simulink model "CAVE_MachE_dSPACE_250912"  (R2024a)
settings: configuration reference "ConfigSetDesktopFixedStep" (kept outside this file)
PreLoadFcn:
  | VSS_BICYCLE=Simulink.Variant('Dual=0');
  | VSS_DUAL=Simulink.Variant('Dual=1');
  | Dual=1;
  | load('DriveCycle2.mat')
PostLoadFcn:
  | if any(exist('dsrtsu_mdlpostloadfcn', 'file') ~= 0), dsrtsu_mdlpostloadfcn('Execute', bdroot); end
InitFcn:
  | , if any(exist('rtifpga_mdlclblib', 'file') ~= 0), rtifpga_mdlclblib('Init', bdroot); end,
  | , if any(exist('dsmpb_private', 'file') ~= 0), dsmpb_private('dsmpb_mdlclblib', 'Init', bdroot); end,
  | load('DriveCycle2.mat')
model workspace (MAT data in the model file):
  Gas = 0.383333333333
values from neighbouring files (symbols this model uses):
  CoastDown =     [Run_Simulink.mat]
  limitedMCT =     [Run_Simulink.mat]
  MCT =     [Run_Simulink.mat]
  pMCT =     [Run_Simulink.mat]
  RealSimPara =     [Run_Simulink.mat]
  Ref_speed = [13 13.007895099 13.015778396 13.023649891 13.031509584 13.039357475 13.047193564 13.055017851 13.062830336 13.070631019 13.0784199 13.086196979 ... (2669 elements, 2669x1)]    [Ref_speed_and_time.mat]
  Ref_time = [0 0.01 0.02 0.03 0.04 0.05 0.06 0.07 0.08 0.09 0.1 0.11 ... (2669 elements, 2669x1)]    [Ref_speed_and_time.mat]
  US06 =     [Run_Simulink.mat]
undefined symbols (not defined in the file or in its folder): AccelCmd, ActTqLF_Nm_, ActTqLR_Nm_, ActTqRF_Nm_, ActTqRR_Nm_, BattChargeLimitMaxPwr, BattChargeLimitSocBpts, BattChargeLimitTbl, BattChrgCapcty, BattDischargeLimitSocBpts, BattDischargeLimitTbl, BattDischargeMaxPwr, BattNumCellsParallel, BattNumCellsSeries, BattOpenVoltCapBpts, BattOpenVoltTbl, BattResistSocBpts, BattResistTbl, BattResistTempBpts, BrakeMaxPrs, BrakeMaxTrq, ChassisDistCg2FrontAxle, ChassisDistCg2RearAxle, ChassisVehMass, CltchCmd, DecelCmd, DiffRatio, DiscIntNeverNeededParam, EnvGravCnst, EnvPrs, EnvTemp, FuelSpecificGrav, GearCmd, h, InitStates, lgSw, MtrEffSpdBpts, MtrEffTbl, MtrEffTrqBpts, MtrPwrMax, MtrTrqMax, SteeringCmd, SupvsryCtrlRegenBrkCutOffTbl, SupvsryCtrlRegenSpdBpts, TestScnrioCycleNum, VEH
libraries: VSIGenLib x122, simulink x112, etargetslib x75, dsmpblib x55, vehdynlibtire x24, CarMaker4SL x20, autolibshared x19, vehdynlibsuspension x14, vehdynlibtirecommon x14, autolibutils x10, VsrLibWheel x8, autolibpowerinfoutils x6
(part 11 of 31)

== system CAVE_MachE_dSPACE_250912/Vehicle Under Test2/Vehicle/Vehicle Dynamics/Vehicle 14DOF/Wheel Routing1 ==
  Info : Inport
  Wheel : Inport  Port=2
  Bus Selector : BusSelector  OutputSignals=InertFrm.FrntAxl.Lft.Disp.Y,InertFrm.FrntAxl.Rght.Disp.Y,InertFrm.RearAxl.Lft.Disp.Y,InertFrm.RearAxl.Rght.Disp.Y
  Bus Selector1 : BusSelector  OutputSignals=InertFrm.FrntAxl.Lft.Disp.X,InertFrm.FrntAxl.Rght.Disp.X,InertFrm.RearAxl.Lft.Disp.X,InertFrm.RearAxl.Rght.Disp.X
  Bus Selector2 : BusSelector  OutputSignals=TireFrame.z,TireFrame.Omega,TireFrame.Kappa,TireFrame.Alpha
  Bus Selector3 : BusSelector  OutputSignals=InertFrm.FrntAxl.Lft.Disp.Z,InertFrm.FrntAxl.Rght.Disp.Z,InertFrm.RearAxl.Lft.Disp.Z,InertFrm.RearAxl.Rght.Disp.Z
  Bus Selector4 : BusSelector  OutputSignals=BdyFrm.FrntAxl.Lft.Disp.z,BdyFrm.FrntAxl.Rght.Disp.z,BdyFrm.RearAxl.Lft.Disp.z,BdyFrm.RearAxl.Rght.Disp.z
  Scope : Scope
  Scope1 : Scope
  Subtract : Sum  Inputs=-+-
  Vector Concatenate{1..4} (4 alike) : Concatenate  NumInputs=4
  Omega : Outport  PortDimensions=4  VectorParamsAs1DForOutWhenUnconnected=off
  Kappa : Outport  Port=2  PortDimensions=4  VectorParamsAs1DForOutWhenUnconnected=off
  Alpha : Outport  Port=3  PortDimensions=4  VectorParamsAs1DForOutWhenUnconnected=off
  XWheel : Outport  Port=4  Unit=m  VectorParamsAs1DForOutWhenUnconnected=off
  YWheel : Outport  Port=5  Unit=m  VectorParamsAs1DForOutWhenUnconnected=off
  ZWheel : Outport  Port=6  PortDimensions=4  VectorParamsAs1DForOutWhenUnconnected=off
  wires:
  Bus Selector4/2 -> Vector Concatenate4/2  "<z>"
  Bus Selector4/3 -> Vector Concatenate4/3  "<z>"
  Bus Selector4/4 -> Vector Concatenate4/4  "<z>"
  Bus Selector4/1 -> Vector Concatenate4/1  "<z>"
  Vector Concatenate4/1 -> Subtract/1
  Vector Concatenate3/1 -> Subtract/2
  Bus Selector3/1 -> Vector Concatenate3/1  "<Z>"
  Bus Selector3/4 -> Vector Concatenate3/4  "<Z>"
  Bus Selector3/3 -> Vector Concatenate3/3  "<Z>"
  Bus Selector3/2 -> Vector Concatenate3/2  "<Z>"
  Info/1 -> Bus Selector/1, Bus Selector3/1, Bus Selector4/1, Bus Selector1/1
  Subtract/1 -> ZWheel/1
  Wheel/1 -> Bus Selector2/1
  Bus Selector2/4 -> Alpha/1  "<Alpha>"
  Bus Selector2/3 -> Kappa/1  "<Kappa>"
  Bus Selector2/2 -> Scope/1, Omega/1  "<Omega>"
  Bus Selector2/1 -> Scope1/1, Subtract/3  "<z>"
  Vector Concatenate2/1 -> XWheel/1
  Bus Selector1/1 -> Vector Concatenate2/1  "<X>"
  Vector Concatenate1/1 -> YWheel/1
  Bus Selector/2 -> Vector Concatenate1/2  "<Y>"
  Bus Selector/3 -> Vector Concatenate1/3  "<Y>"
  Bus Selector1/2 -> Vector Concatenate2/2  "<X>"
  Bus Selector/4 -> Vector Concatenate1/4  "<Y>"
  Bus Selector1/3 -> Vector Concatenate2/3  "<X>"
  Bus Selector/1 -> Vector Concatenate1/1  "<Y>"
  Bus Selector1/4 -> Vector Concatenate2/4  "<X>"

== system CAVE_MachE_dSPACE_250912/Vehicle Under Test2/Vehicle/Vehicle Dynamics/Vehicle 14DOF/Wheels and Tires ==
  Suspension : Inport
  Axle Torque : Inport  Port=2
  Brake Press : Inport  Port=3  Unit=Pa
  Ground Input : Inport  Port=4
  Friction : Inport  Port=5  PortDimensions=4
  Bus Selector1 : BusSelector  OutputSignals=Whl.Ang,Whl.F,Whl.AngVel,Whl.xdot,Whl.ydot
  Constant3 : Constant  Value=zeros(4,1)
  Cont LPF : autolibutils/Cont LPF  wc=100*2*pi  AbsoluteTolerance=auto  aMode=2
  Cont LPF1 : autolibutils/Cont LPF  wc=100*2*pi  AbsoluteTolerance=auto  aMode=2
  Manual Switch6 : ManualSwitch
  Matrix Concatenate : Concatenate  NumInputs=3  Mode=Multidimensional array
  Reshape1 : Reshape
  Reshape2 : Reshape
  Saturation : Saturate  UpperLimit=10*9.81*2040  LowerLimit=-10*9.81*2040  ZeroCross=off
  Selector : Selector  NumberOfDimensions=2  InputPortWidth=3  IndexOptions=Index vector (dialog),Select all  Indices=[3],1  OutputSizes=1,1
  Selector1 : Selector  NumberOfDimensions=2  InputPortWidth=1  IndexOptions=Index vector (dialog),Select all  Indices=[3],1  OutputSizes=1,1
  Selector2 : Selector  NumberOfDimensions=2  InputPortWidth=3  IndexOptions=Index vector (dialog),Select all  Indices=3,1  OutputSizes=1,1
  Selector3 : Selector  NumberOfDimensions=2  InputPortWidth=3  IndexOptions=Index vector (dialog),Select all  Indices=1,1  OutputSizes=1,1
  Terminator{,1,3..5} (5 alike) : Terminator
  VDBS : Subsystem  VariantControl=0
  Wheels : Outport  VectorParamsAs1DForOutWhenUnconnected=off
  wires:
  VDBS/1(Wheels) -> Wheels/1  "Wheels"
  Bus Selector1/2 -> Selector/1  "<F>"
  VDBS/2(FrntAxlF) -> Terminator/1
  VDBS/3(RearAxlF) -> Terminator1/1
  VDBS/4(Omega) -> Terminator3/1
  VDBS/5(Mz) -> Terminator4/1
  Selector1/1 -> Reshape1/1
  Matrix Concatenate/1 -> VDBS/7(VehVel)
  Axle Torque/1 -> VDBS/3(AxleTrq)
  Selector2/1 -> VDBS/1(WheelAng)  "Wheel Angles"
  Constant3/1 -> Manual Switch6/1
  Manual Switch6/1 -> VDBS/2(CamberAng)  "Camber Angles"
  Selector/1 -> Reshape2/1
  Saturation/1 -> VDBS/5(Fz)
  Ground Input/1 -> VDBS/8(Ground Level)
  VDBS/7(SuspWhlVz) -> Matrix Concatenate/3  "zdot"
  Bus Selector1/1 -> Cont LPF1/1  "<Ang>"
  Selector3/1 -> Manual Switch6/2  "Camber Angles"
  Suspension/1 -> Bus Selector1/1
  Bus Selector1/4 -> Matrix Concatenate/1  "<xdot>"
  Bus Selector1/5 -> Matrix Concatenate/2  "<ydot>"
  VDBS/6(SuspWhlPz) -> Terminator5/1  "z"
  Reshape2/1 -> Cont LPF/1
  Bus Selector1/3 -> Selector1/1  "<AngVel>"
  Reshape1/1 -> VDBS/6(r)
  Brake Press/1 -> VDBS/4(BrkPrs)
  Friction/1 -> VDBS/9(Friction)
  Cont LPF/1 -> Saturation/1
  Cont LPF1/1 -> Selector3/1, Selector2/1

== system CAVE_MachE_dSPACE_250912/Vehicle Under Test2/Vehicle/Vehicle Dynamics/Vehicle 7DOF/Brake Pressure ==
  BrkReq : Inport
  Bus Creator1 : BusCreator  Inputs=2
  Gain : Gain  Gain=BrakeMaxPrs
  Gain{1..4} (4 alike) : Gain  Gain=0.5
  Saturation{,1..3} (4 alike) : Saturate  UpperLimit=BrakeMaxPrs  LowerLimit=0  ZeroCross=off
  Signal Specification : SignalSpecification  Unit=Pa
  Terminator : Terminator
  Vector Concatenate2 : Concatenate  NumInputs=4
  BrakePrs : Outport  Unit=Pa
  wires:
  BrkReq/1 -> Gain/1, Bus Creator1/1  "BrkReq"
  Gain/1 -> Signal Specification/1
  Signal Specification/1 -> Gain2/1, Gain1/1, Bus Creator1/2  "BrkPrs"
  Bus Creator1/1 -> Terminator/1  "WhlBrk"
  Gain1/1 -> Gain4/1
  Gain2/1 -> Gain3/1
  Gain3/1 -> Saturation/1, Saturation1/1
  Gain4/1 -> Saturation2/1, Saturation3/1
  Vector Concatenate2/1 -> BrakePrs/1
  Saturation/1 -> Vector Concatenate2/1
  Saturation1/1 -> Vector Concatenate2/2
  Saturation2/1 -> Vector Concatenate2/3
  Saturation3/1 -> Vector Concatenate2/4

== system CAVE_MachE_dSPACE_250912/Vehicle Under Test2/Vehicle/Vehicle Dynamics/Vehicle 7DOF/Longitudinal Wheels 4DOF ==
  WhlAng : Inport
  AxlTrq : Inport  Port=2
  BrkPrs : Inport  Port=3
  Gnd : Inport  Port=4  PortDimensions=4
  lam_mu : Inport  Port=5  PortDimensions=4
  VehFdbk : Inport  Port=6
  Axle Forces : Subsystem  Variant=on  VariantControlMode=label  LabelModeActiveChoice=1
  Bus Selector5 : BusSelector  OutputSignals=BdyFrm.Cg.AngVel.r
  Constant : vehdynlibtirecommon/Constant  const=220000  numWheels=4
  Constant3 : vehdynlibtirecommon/Constant  const=0  numWheels=4
  Terminator2 : Terminator
  Tire2Veh : Subsystem
  Tires : Subsystem
  Veh2Tire : Subsystem
  Velocity and Vertical Load : Subsystem  Variant=on  VariantControlMode=label  LabelModeActiveChoice=1
  Wheel Angles : Subsystem
  FrntAxlF : Outport  Unit=N  VectorParamsAs1DForOutWhenUnconnected=off
  RearAxlF : Outport  Port=2  Unit=N  VectorParamsAs1DForOutWhenUnconnected=off
  Omega : Outport  Port=3  VectorParamsAs1DForOutWhenUnconnected=off
  Kappa : Outport  Port=4  VectorParamsAs1DForOutWhenUnconnected=off
  Alpha : Outport  Port=5  VectorParamsAs1DForOutWhenUnconnected=off
  zAxle : Outport  Port=6  VectorParamsAs1DForOutWhenUnconnected=off
  wires:
  Wheel Angles/1(WhlAngB) -> Veh2Tire/5(WhlAng)
  Tires/1(Wheel) -> Tire2Veh/1(Wheel)
  lam_mu/1 -> Tires/9(lam_mu)
  Constant/1 -> Tires/7(TirePrs)
  Constant3/1 -> Wheel Angles/2(Camber), Tires/6(Camber)
  Veh2Tire/3(xdotAxle) -> Tires/3(Vx)  "Vx"
  Gnd/1 -> Tires/10(Gnd)
  VehFdbk/1 -> Bus Selector5/1, Velocity and Vertical Load/1(VehFdbk)
  AxlTrq/1 -> Veh2Tire/1(AxlTrq)
  Veh2Tire/1(T) -> Tires/1(AxlTrq)
  Veh2Tire/2(P) -> Tires/2(BrkPrs)
  BrkPrs/1 -> Veh2Tire/2(BrkPrs)
  Bus Selector5/1 -> Veh2Tire/3(r)  "<r>"
  Veh2Tire/6(zdotAxle) -> Terminator2/1
  WhlAng/1 -> Wheel Angles/1(WheelAng)  "FrontWheelAngles"
  Veh2Tire/4(ydotAxle) -> Tires/4(Vy)  "Vy"
  Veh2Tire/5(psidot) -> Tires/5(r)
  Velocity and Vertical Load/2(Fz) -> Tires/8(Fz)
  Velocity and Vertical Load/1(VehVel) -> Veh2Tire/4(VehVel)
  Axle Forces/1(FrntAxlF) -> FrntAxlF/1
  Axle Forces/2(RearAxlF) -> RearAxlF/1
  Tire2Veh/1(FwF) -> Axle Forces/1(F)
  Tire2Veh/2(FwR) -> Axle Forces/2(R)
  Tire2Veh/3(z) -> zAxle/1
  Tire2Veh/4(Omega) -> Omega/1
  Tire2Veh/5(Kappa) -> Kappa/1
  Tire2Veh/6(Alpha) -> Alpha/1

== system CAVE_MachE_dSPACE_250912/Vehicle Under Test2/Vehicle/Vehicle Dynamics/Vehicle 7DOF/RototestDummy ==
  Bus Creator1 : BusCreator  Inputs=ActTqLF_Nm_,ActTqRF_Nm_,ActTqLR_Nm_,ActTqRR_Nm_
  Bus Creator2 : BusCreator  Inputs=Car Trq_T2WFL,Car Trq_T2WFR,Car Trq_T2WRL,Car Trq_T2WRR
  Bus Creator3 : BusCreator  Inputs=1
  Bus Creator4 : BusCreator  Inputs=1
  Bus Selector14 : BusSelector  OutputSignals=VehSpd
  Bus Selector15 : BusSelector  OutputSignals=TireFrame.Fx
  Constant{1..14} (14 alike) : Constant  Value=0
  Vector Concatenate3 : Concatenate  NumInputs=4
  CarTrqT2W : Outport
  AxleTrq : Outport  Port=2
  BrakePressed_flag : Outport  Port=3
  <VehSpd> : Outport  Port=4
  <Fx> : Outport  Port=5
  wires:
  Constant10/1 -> Bus Selector14/1  "VehSpd"
  Bus Creator4/1 -> Bus Creator3/1  "TireFrame"
  Bus Creator1/1 -> AxleTrq/1  "AxleTrq"
  Constant9/1 -> Bus Creator1/4  "ActTqRR_Nm_"
  Constant13/1 -> Bus Creator2/3  "CarTrq_T2WRL"
  Constant4/1 -> Vector Concatenate3/4
  Bus Creator3/1 -> Bus Selector15/1
  Vector Concatenate3/1 -> Bus Creator4/1  "Fx"
  Constant3/1 -> Vector Concatenate3/3
  Constant2/1 -> Vector Concatenate3/2
  Constant14/1 -> Bus Creator2/4  "CarTrq_T2WRR"
  Constant6/1 -> Bus Creator1/1  "ActTqLF_Nm_"
  Constant1/1 -> Vector Concatenate3/1
  Constant8/1 -> Bus Creator1/3  "ActTqLR_Nm_"
  Constant11/1 -> Bus Creator2/1  "CarTrq_T2WFL"
  Constant7/1 -> Bus Creator1/2  "ActTqRF_Nm_"
  Constant12/1 -> Bus Creator2/2  "CarTrq_T2WFR"
  Bus Creator2/1 -> CarTrqT2W/1  "CarTrqT2W"
  Bus Selector14/1 -> <VehSpd>/1  "<VehSpd>"
  Constant5/1 -> BrakePressed_flag/1  "BrakePressed_flag"
  Bus Selector15/1 -> <Fx>/1  "<Fx>"

== system CAVE_MachE_dSPACE_250912/Vehicle Under Test2/Vehicle/Vehicle Dynamics/Vehicle 7DOF/Steering ==
  SteeringCmd : Inport
  Ground : Ground
  Kinematic Steering : vehdynlibsteering/Kinematic Steering  StrgType=Ackerman  StrgRatioType=Constant  Loc=Front  NrmlFctr=1  TrckWdth=1.9  WhlBase=ChassisDistCg2FrontAxle+ChassisDistCg2RearAxle  Db=0  StrgRng=3*pi  StrgAngBpts="[-6.2832   -5.0265   -3.7699   -2.5133   -1.2566         0    1.2566    2.5133    3.7699    5.0265    6.2832]"  StrgRatioTbl=|  StrgRatio=18  PctAckIn=off  PctAck=100  PctAckTbl=ones(1,11)*100  StrgArmLngth=0.1  RckCsLngth=0.5  TieRodLngth=0.248  D=0.2  PnnRadius=0.0057  PnnRadiusTbl="[0.0055    0.0055    0.0056    0.0057    0.0058    0.0057    0.0057    0.0057    0.0056    0.0055    0.0055]"  RodLngth=0.1  ParaArmLngth=0.9  aMode=2
      | [13.5000   13.3750   13.2500   13.1250   13.0000   13.0000   13.0000   13.1250   13.2500   13.3750   13.5000
      | ]
  Terminator1 : Terminator
  Vector Concatenate : Concatenate
  Vector Concatenate1 : Concatenate
  Vector Concatenate2 : Concatenate
  WhlAng : Outport  Unit=rad
  wires:
  Kinematic Steering/1 -> Terminator1/1
  Vector Concatenate2/1 -> WhlAng/1
  Kinematic Steering/2 -> Vector Concatenate/1
  Vector Concatenate1/1 -> Vector Concatenate2/2  "RearWheelAngles"
  Vector Concatenate/1 -> Vector Concatenate2/1  "FrontWheelAngles"
  Ground/1 -> Vector Concatenate1/2, Vector Concatenate1/1
  Kinematic Steering/3 -> Vector Concatenate/2
  SteeringCmd/1 -> Kinematic Steering/1

== system CAVE_MachE_dSPACE_250912/Vehicle Under Test2/Vehicle/Vehicle Dynamics/Vehicle 7DOF/Subsystem4 ==
  Cgxyzdot : Inport
  CgXYZ : Inport  Port=2
  CgXYZdot : Inport  Port=3
  angles : Inport  Port=4
  pqr : Inport  Port=5
  Cgaxyz : Inport  Port=6
  Beta : Inport  Port=7
  GeomXYZ : Inport  Port=8
  GeomXYZdot : Inport  Port=9
  Omega : Inport  Port=10
  Kappa : Inport  Port=11
  Alpha : Inport  Port=12
  XWheel : Inport  Port=13
  YWheel : Inport  Port=14
  dzWheel : Inport  Port=15
  Bus Creator : BusCreator  Inputs=26
  Bus Creator3 : BusCreator  Inputs=6
  Demux{,1..7} (8 alike) : Demux  Outputs=3
  Subsystem : Subsystem
  Chassis : Outport  VectorParamsAs1DForOutWhenUnconnected=off
  Wheels : Outport  Port=2  VectorParamsAs1DForOutWhenUnconnected=off
  wires:
  Bus Creator/1 -> Chassis/1  "Chassis"
  Omega/1 -> Bus Creator3/3  "Omega"
  dzWheel/1 -> Bus Creator3/6  "dZWheel"
  Kappa/1 -> Bus Creator3/1  "Kappa"
  Bus Creator3/1 -> Wheels/1  "Wheels"
  YWheel/1 -> Bus Creator3/5  "YWheel"
  XWheel/1 -> Bus Creator3/4  "XWheel"
  Alpha/1 -> Bus Creator3/2  "Alpha"
  Cgxyzdot/1 -> Demux/1
  CgXYZ/1 -> Demux1/1
  CgXYZdot/1 -> Subsystem/1(CgXYZdot), Demux2/1
  angles/1 -> Subsystem/2(angles), Demux3/1
  pqr/1 -> Demux4/1
  Cgaxyz/1 -> Demux5/1
  GeomXYZdot/1 -> Demux7/1
  GeomXYZ/1 -> Demux6/1
  Demux/1 -> Bus Creator/1  "xdot"
  Demux/2 -> Bus Creator/2  "ydot"
  Demux/3 -> Bus Creator/3  "zdot"
  Demux1/1 -> Bus Creator/4  "X"
  Demux1/2 -> Bus Creator/5  "Y"
  Demux1/3 -> Bus Creator/6  "Z"
  Demux2/1 -> Bus Creator/7  "Xdot"
  Demux2/2 -> Bus Creator/8  "Ydot"
  Demux2/3 -> Bus Creator/9  "Zdot"
  Demux3/1 -> Bus Creator/10  "phi"
  Demux3/2 -> Bus Creator/11  "theta"
  Demux3/3 -> Bus Creator/12  "psi"
  Demux4/1 -> Bus Creator/13  "p"
  Demux4/2 -> Bus Creator/14  "q"
  Demux4/3 -> Bus Creator/15  "r"
  Demux5/1 -> Bus Creator/16  "ax"
  Demux5/2 -> Bus Creator/17  "ay"
  Demux5/3 -> Bus Creator/18  "az"
  Beta/1 -> Bus Creator/19  "Beta"
  Demux6/1 -> Bus Creator/20  "GeomX"
  Demux6/2 -> Bus Creator/21  "GeomY"
  Demux6/3 -> Bus Creator/22  "GeomZ"
  Demux7/1 -> Bus Creator/23  "GeomXdot"
  Demux7/2 -> Bus Creator/24  "GeomYdot"
  Demux7/3 -> Bus Creator/25  "GeomZdot"
  Subsystem/1(VehSpd) -> Bus Creator/26  "VehSpd"

== system CAVE_MachE_dSPACE_250912/Vehicle Under Test2/Vehicle/Vehicle Dynamics/Vehicle 7DOF/Vehicle Body 3DOF External Longitudinal Wheels ==
  WhlAng : Inport
  "FwF " : Inport  Port=2
  "FwR " : Inport  Port=3
  WindXYZ : Inport  Port=4
  Friction : Inport  Port=5  Unit=1  PortDimensions=4
  Bicycle : Subsystem  VariantControl=0
  Dual : Subsystem  VariantControl=1
  " Info" : Outport  VectorParamsAs1DForOutWhenUnconnected=off
  " XWheel" : Outport  Port=2  VectorParamsAs1DForOutWhenUnconnected=off
  " YWheel" : Outport  Port=3  VectorParamsAs1DForOutWhenUnconnected=off

== system CAVE_MachE_dSPACE_250912/Vehicle Under Test2/Vehicle/Vehicle Dynamics/Vehicle Longitudinal/Brake Pressure ==
  BrkReq : Inport
  Bus Creator1 : BusCreator  Inputs=2
  Gain : Gain  Gain=BrakeMaxPrs
  Gain{1..4} (4 alike) : Gain  Gain=0.5
  Saturation{,1..3} (4 alike) : Saturate  UpperLimit=BrakeMaxPrs  LowerLimit=0  ZeroCross=off
  Signal Specification : SignalSpecification  Unit=Pa
  Terminator : Terminator
  Vector Concatenate2 : Concatenate  NumInputs=4
  BrakePrs : Outport  Unit=Pa
  wires:
  BrkReq/1 -> Gain/1, Bus Creator1/1  "BrkReq"
  Gain/1 -> Signal Specification/1
  Signal Specification/1 -> Gain2/1, Gain1/1, Bus Creator1/2  "BrkPrs"
  Bus Creator1/1 -> Terminator/1  "WhlBrk"
  Gain1/1 -> Gain4/1
  Gain2/1 -> Gain3/1
  Gain3/1 -> Saturation/1, Saturation1/1
  Gain4/1 -> Saturation2/1, Saturation3/1
  Vector Concatenate2/1 -> BrakePrs/1
  Saturation/1 -> Vector Concatenate2/1
  Saturation1/1 -> Vector Concatenate2/2
  Saturation2/1 -> Vector Concatenate2/3
  Saturation3/1 -> Vector Concatenate2/4

== system CAVE_MachE_dSPACE_250912/Vehicle Under Test2/Vehicle/Vehicle Dynamics/Vehicle Longitudinal/Longitudinal Wheels ==
  BrkPrs : Inport
  AxleTorq : Inport  Port=2
  Bus Creator : BusCreator  Inputs=3
  Bus Selector : BusSelector  OutputSignals=WhlRearInfo,Omega3,Omega4
  Bus Selector1 : BusSelector  OutputSignals=WhlFrontInfo,Omega1,Omega2
  Front Diff Wheels : Subsystem
  Rear Wheels : Subsystem
  Vector Concatenate : Concatenate  NumInputs=4
  FrontAxle : PMIOPort  Side=Right
  RearAxle : PMIOPort  Port=2  Side=Right
  Whl : Outport
  wires:
  Rear Wheels/1(Info) -> Bus Selector/1  "WhlRearInfo"
  Front Diff Wheels/1(Info) -> Bus Selector1/1  "WhlFrontInfo"
  Bus Creator/1 -> Whl/1  "Whl"
  BrkPrs/1 -> Front Diff Wheels/1(BrkPrs), Rear Wheels/1(BrkPrs)
  AxleTorq/1 -> Front Diff Wheels/2(AxleTorq)
  Bus Selector/2 -> Vector Concatenate/3  "<Omega3>"
  Bus Selector1/1 -> Bus Creator/1  "<WhlFrontInfo>"
  Bus Selector1/2 -> Vector Concatenate/1  "<Omega1>"
  Bus Selector1/3 -> Vector Concatenate/2  "<Omega2>"
  Bus Selector/3 -> Vector Concatenate/4  "<Omega4>"
  Bus Selector/1 -> Bus Creator/2  "<WhlRearInfo>"
  Vector Concatenate/1 -> Bus Creator/3  "Omega"
  connections:
  RearAxle/RConn1 -- Rear Wheels/RConn1
  Front Diff Wheels/RConn1 -- FrontAxle/RConn1

== system CAVE_MachE_dSPACE_250912/Vehicle Under Test2/Vehicle/Vehicle Dynamics/Vehicle Longitudinal/RototestDummy ==
  Bus Creator1 : BusCreator  Inputs=ActTqLF_Nm_,ActTqRF_Nm_,ActTqLR_Nm_,ActTqRR_Nm_
  Bus Creator2 : BusCreator  Inputs=Car Trq_T2WFL,Car Trq_T2WFR,Car Trq_T2WRL,Car Trq_T2WRR
  Bus Creator3 : BusCreator  Inputs=1
  Bus Creator4 : BusCreator  Inputs=1
  Bus Selector14 : BusSelector  OutputSignals=VehSpd
  Bus Selector15 : BusSelector  OutputSignals=TireFrame.Fx
  Constant{1..14} (14 alike) : Constant  Value=0
  Vector Concatenate3 : Concatenate  NumInputs=4
  CarTrqT2W : Outport
  AxleTrq : Outport  Port=2
  BrakePressed_flag : Outport  Port=3
  <VehSpd> : Outport  Port=4
  <Fx> : Outport  Port=5
  wires:
  Constant10/1 -> Bus Selector14/1  "VehSpd"
  Bus Creator4/1 -> Bus Creator3/1  "TireFrame"
  Bus Creator1/1 -> AxleTrq/1  "AxleTrq"
  Constant9/1 -> Bus Creator1/4  "ActTqRR_Nm_"
  Constant13/1 -> Bus Creator2/3  "CarTrq_T2WRL"
  Constant4/1 -> Vector Concatenate3/4
  Bus Creator3/1 -> Bus Selector15/1
  Vector Concatenate3/1 -> Bus Creator4/1  "Fx"
  Constant3/1 -> Vector Concatenate3/3
  Constant2/1 -> Vector Concatenate3/2
  Constant14/1 -> Bus Creator2/4  "CarTrq_T2WRR"
  Constant6/1 -> Bus Creator1/1  "ActTqLF_Nm_"
  Constant1/1 -> Vector Concatenate3/1
  Constant8/1 -> Bus Creator1/3  "ActTqLR_Nm_"
  Constant11/1 -> Bus Creator2/1  "CarTrq_T2WFL"
  Constant7/1 -> Bus Creator1/2  "ActTqRF_Nm_"
  Constant12/1 -> Bus Creator2/2  "CarTrq_T2WFR"
  Bus Creator2/1 -> CarTrqT2W/1  "CarTrqT2W"
  Bus Selector14/1 -> <VehSpd>/1  "<VehSpd>"
  Constant5/1 -> BrakePressed_flag/1  "BrakePressed_flag"
  Bus Selector15/1 -> <Fx>/1  "<Fx>"

== system CAVE_MachE_dSPACE_250912/Vehicle Under Test2/Vehicle/Vehicle Dynamics/Vehicle Longitudinal/Vehicle Body ==
  RoadGrade : Inport
  WindX : Inport  Port=2
  Logitudinal Vehicle Body : Subsystem
  Subsystem1 : Subsystem
      mask Display: disp('')
  FrontAxle : PMIOPort  Side=Left
  RearDiff : PMIOPort  Port=2  Side=Left
  Chassis : Outport
  wires:
  Logitudinal Vehicle Body/1(VehSpd) -> Subsystem1/1(VehSpd)
  Logitudinal Vehicle Body/2(VehDist) -> Subsystem1/2(VehDist)
  Logitudinal Vehicle Body/3(FrontAxleFrc) -> Subsystem1/3(FrontAxleFrc)
  Logitudinal Vehicle Body/4(RearAxleFrc) -> Subsystem1/4(RearAxleFrc)
  Subsystem1/1(ChassisPlant) -> Chassis/1
  RoadGrade/1 -> Logitudinal Vehicle Body/1(RoadGrade)
  WindX/1 -> Logitudinal Vehicle Body/2(WindVel)
  connections:
  RearDiff/RConn1 -- Logitudinal Vehicle Body/LConn2
  FrontAxle/RConn1 -- Logitudinal Vehicle Body/LConn1

== system CAVE_MachE_dSPACE_250912/Vehicle Under Test3/Vehicle/Actuation and Outputs/MOOG Brake Actuator/ CAN Settings ==
  " CAN diagnostic Counter" : Subsystem  mask{TimeOutDuration=0.1}
      mask prompts: TimeOutDuration "CAN Time Out Duration"
  Data Type Conversion1 : DataTypeConversion  SaturateOnIntegerOverflow=off  RndMeth=Floor
  Data Type Conversion3 : DataTypeConversion  SaturateOnIntegerOverflow=off  RndMeth=Floor
  "RPDO3 Enable " : Constant
  RPDO3 period : Constant  Value=0.001
  RPDO3\PDU Features\PDU Cyclic Timing Control\RPDO3 Timing Control Period [BrakeAct_Config\Simulated ECUs\CANOpen_MOOG_02\Controller\TX\PDUs] : dsmpblib/Data Outport  Priority=-10000
      settings: SourceProductName=dSPACE Model Interface Package for Simulink (MIPS)
  RPDO3\PDU Features\PDU Enable\RPDO3 Enable [BrakeAct_Config\Simulated ECUs\CANOpen_MOOG_02\Controller\TX\PDUs] : dsmpblib/Data Outport  Priority=-10000
      settings: SourceProductName=dSPACE Model Interface Package for Simulink (MIPS)
  TPDO3\PDU Features\PDU RX Status\TPDO3 Counter [BrakeAct_Config\Simulated ECUs\CANOpen_MOOG_02\Controller\RX\PDUs] : dsmpblib/Data Inport  Priority=10000
      settings: SourceProductName=dSPACE Model Interface Package for Simulink (MIPS)
  CAN_CommsOK_Flg : Outport
  wires:
  "RPDO3 Enable "/1 -> Data Type Conversion3/1
  Data Type Conversion3/1 -> RPDO3\PDU Features\PDU Enable\RPDO3 Enable [BrakeAct_Config\Simulated ECUs\CANOpen_MOOG_02\Controller\TX\PDUs]/1
  RPDO3 period/1 -> RPDO3\PDU Features\PDU Cyclic Timing Control\RPDO3 Timing Control Period [BrakeAct_Config\Simulated ECUs\CANOpen_MOOG_02\Controller\TX\PDUs]/1
  TPDO3\PDU Features\PDU RX Status\TPDO3 Counter [BrakeAct_Config\Simulated ECUs\CANOpen_MOOG_02\Controller\RX\PDUs]/1 -> Data Type Conversion1/1
  Data Type Conversion1/1 -> " CAN diagnostic Counter"/1(RX Counter)
  " CAN diagnostic Counter"/1(CommsOKFlag) -> CAN_CommsOK_Flg/1  "TPDO3_CommsOK_Flg"

== system CAVE_MachE_dSPACE_250912/Vehicle Under Test3/Vehicle/Actuation and Outputs/MOOG Brake Actuator/MOOG Interface ==
  note: RAV4
      | Min an Max stops need adjusting otherwise:
      | - brake lights come on at 13% (with ajustment, it comes on at 2-3%
      | - 100% pedal can cause the actuator to generate a fault (maybe over current)
      | Min Offset +5500
      | Max Offset -5500
      |
      | Mach-e
      | Min Offset +5500
      | Max Offset -3500
      | this results in brake lights coming on at 4% and off at 1%
      |
      | total travel needs to be more than 35000 for valid range,
      | otherwise, brake booster was most likely not active
  CAN_CommsOK_Flg : Inport
  TargetPosition [pct] : Inport  Port=2
  StatusWord in : Inport  Port=3
  ActualPosition_cnt in : Inport  Port=4
  Mode of operation in : Inport  Port=5
  ActuatorMinTravelForReady : Constant  Value=35000
  Bus Creator : BusCreator  Inputs=2
  Constant1 : Constant  Value=100
  Constant2 : Constant  Value=100
  Data Type Conversion : DataTypeConversion  SaturateOnIntegerOverflow=off  RndMeth=Floor
  Data Type Conversion1 : DataTypeConversion  SaturateOnIntegerOverflow=off  RndMeth=Floor
  Display{2..5} (4 alike) : Display
  Gain : Gain
  Gain1 : Gain
  Gain2 : Gain
  MOOG State Machine : Stateflow chart  TreatAsAtomicUnit=on
  Max Stop Adjustment : Subsystem  TreatAsAtomicUnit=on
  Memory : Memory  InheritSampleTime=on
  Memory1 : Memory  InheritSampleTime=on
  Memory2 : Memory  InheritSampleTime=on
  Min Stop Adjustment : Subsystem  TreatAsAtomicUnit=on
  MoogResetCmd : Constant  Value=0
  PositionLearningTrigger : Constant  Value=0
  Product : Product  Inputs=*/*
  Product1 : Product  Inputs=*/*
  Rising edge : Subsystem
  Rising edge1 : Subsystem
  Sum : Sum  Inputs=|+-
  Sum1 : Sum  Inputs=|++
  Sum2 : Sum  Inputs=|+-
  Terminator1 : Terminator
  Commands : Outport
  ActualPosition [pct] : Outport  Port=2
  BrakeActuatorReady : Outport  Port=3
  wires:
  Sum1/1 -> MOOG State Machine/6(TargetPosition_cnt)  "TargetPosition_cnt"
  Bus Creator/1 -> Commands/1
  [MaxStop_cnt] -> Sum/1
  [MinStop_cnt] -> Sum/2
  MOOG State Machine/1(ControlWord) -> Bus Creator/1  "ControlWord"
  MOOG State Machine/3(Actuator_Ready) -> BrakeActuatorReady/1  "Actuator_Ready"
  MOOG State Machine/4(FaultCntr) -> Display2/1  "FaultCounter"
  Sum/1 -> Product1/2, Product/3
  TargetPosition [pct]/1 -> Product/1  "TargetPosition_pct"
  Constant2/1 -> Product/2
  Gain/1 -> Data Type Conversion1/1, Sum2/1
  Gain1/1 -> Terminator1/1  "Mode of operation"
  Product/1 -> Sum1/1
  [MinStop_cnt] -> Sum2/2
  Sum2/1 -> Product1/1
  Constant1/1 -> Product1/3
  Product1/1 -> ActualPosition [pct]/1  "ActualPosition_pct"
  StatusWord in/1 -> Data Type Conversion/1
  Data Type Conversion/1 -> MOOG State Machine/4(StatusWord)  "StatusWord"
  ActualPosition_cnt in/1 -> Gain/1
  Mode of operation in/1 -> Gain1/1
  MOOG State Machine/5(MoogSMState) -> Display3/1  "MoogSMState"
  MOOG State Machine/6(InitComplete) -> Display4/1  "InitComplete"
  MOOG State Machine/7(MoogOpMode) -> Display5/1  "MoogOpMode"
  MOOG State Machine/10(MinStop) -> Memory1/1  "MinStop"
  MOOG State Machine/9(MaxStop) -> Memory/1  "MaxStop"
  MOOG State Machine/8(LearningComplete) -> Memory2/1  "LearningComplete"
  MOOG State Machine/2(PositionCmd) -> Gain2/1
  Gain2/1 -> Bus Creator/2  "TargetPositionFinal_cnt"
  Data Type Conversion1/1 -> MOOG State Machine/5(ActualPosition_cnt)  "ActualPosition_cnt"
  MoogResetCmd/1 -> Rising edge/1(In)
  Rising edge/1(Out) -> MOOG State Machine/2(ResetCmd)
  PositionLearningTrigger/1 -> Rising edge1/1(In)
  Rising edge1/1(Out) -> MOOG State Machine/3(PositionLearningTrigger)
  Max Stop Adjustment/1(Out1) -> [MaxStop_cnt]  "MaxStop_cnt"
  Min Stop Adjustment/1(Out1) -> [MinStop_cnt]  "MinStop_cnt"
  [MinStop_cnt] -> Sum1/2
  Memory/1 -> Max Stop Adjustment/1(In1)
  Memory1/1 -> Min Stop Adjustment/1(In1)
  Memory2/1 -> Max Stop Adjustment/Enable, Min Stop Adjustment/Enable
  CAN_CommsOK_Flg/1 -> MOOG State Machine/1(CAN_CommsOK_Flg)
  ActuatorMinTravelForReady/1 -> MOOG State Machine/7(ActuatorMinTravelForReady)

== system CAVE_MachE_dSPACE_250912/Vehicle Under Test3/Vehicle/Battery/Battery/Lithium Ion Battery Pack1 ==
  note: Info
  BattCurr : Inport  Unit=A
  BattTemp : Inport  Port=2  Unit=K
  Datasheet Battery Internal : Subsystem  AncestorBlock=autolibbatterycommon/Datasheet Battery Internal
  Info Bus : autolibbatterycommon/Info  RefBlkName='autolibdatasheetbattery/Datasheet Battery'
  Output Passthrough : autolibbatterycommon/Output Passthrough  SystemSampleTime=-1  VariantActivationTime=update diagram  AllowFlexibleInterface=on  Latency=0  AutoFrameSizeCalculation=off
  Info : Outport  VectorParamsAs1DForOutWhenUnconnected=off
  BattVolt : Outport  Port=2  Unit=V  VectorParamsAs1DForOutWhenUnconnected=off
  wires:
  [BattPwrLoss] -> Info Bus/5
  Output Passthrough/1 -> BattVolt/1, [BattVolt]
  [BattVolt] -> Info Bus/4
  Datasheet Battery Internal/1(LdCurrFeed) -> [LdCurrFeed]
  [LdCurrFeed] -> Info Bus/3
  Datasheet Battery Internal/5(BattPwrLoss) -> [BattPwrLoss]
  Datasheet Battery Internal/2(OutVoltUnfilt) -> Output Passthrough/1
  Datasheet Battery Internal/3(LdAmpHr) -> [LdAmpHr]
  Datasheet Battery Internal/4(BattSoc) -> [BattSoc]
  BattTemp/1 -> Datasheet Battery Internal/2(BattTemp)
  BattCurr/1 -> Datasheet Battery Internal/1(BattCurr)
  Info Bus/1 -> Info/1
  [BattSoc] -> Info Bus/2
  [LdAmpHr] -> Info Bus/1

== system CAVE_MachE_dSPACE_250912/Vehicle Under Test3/Vehicle/Driver and Drive Cycle/Driver and PI with FF Control/Speed controller set ==
  RefSpd [km/hr] : Inport
  VehSpd : Inport  Port=2
  Control selection : Constant
  In-house CAVE : Subsystem  VariantControl=varaint1
  Multiport Switch1 : MultiPortSwitch  SaturateOnIntegerOverflow=off  InputSameDT=off
  Multiport Switch2 : MultiPortSwitch  SaturateOnIntegerOverflow=off  InputSameDT=off
  Multiport Switch3 : MultiPortSwitch  SaturateOnIntegerOverflow=off  InputSameDT=off
  PIF : Subsystem  VariantControl=varaint2
  Predictive : Subsystem  VariantControl=varaint3
  Scope : Scope  NumInputPorts=2
  Speed tracking controller : Subsystem  Commented=on  Variant=on  VariantControlMode=label  VariantControl=Variant1  LabelModeActiveChoice=varaint1  PropagateVariantConditions=on
  Out1 : Outport
  Out2 : Outport  Port=2
  Out3 : Outport  Port=3
  wires:
  Control selection/1 -> Multiport Switch3/1, Multiport Switch2/1, Multiport Switch1/1
  RefSpd [km/hr]/1 -> Scope/1, In-house CAVE/1(RefSpd [km/hr]), Predictive/1(RefSpd [km/hr]), PIF/1(RefSpd [km/hr])
  In-house CAVE/1(AccelPedalCmd) -> Multiport Switch1/2
  PIF/1(AccelPedalCmd) -> Multiport Switch1/3
  Predictive/1(AccelPedalCmd) -> Multiport Switch1/4
  In-house CAVE/2(BrakePedalCmd) -> Multiport Switch2/2
  PIF/2(BrakePedalCmd) -> Multiport Switch2/3
  Predictive/2(BrakePedalCmd) -> Multiport Switch2/4
  In-house CAVE/3(Out3) -> Multiport Switch3/2
  PIF/3(Out3) -> Multiport Switch3/3
  Predictive/3(Out3) -> Multiport Switch3/4
  Multiport Switch3/1 -> Out3/1  "BrakeSwitch"
  Multiport Switch2/1 -> Out2/1  "BrakePedalCmd"
  Multiport Switch1/1 -> Out1/1  "AccelPedalCmd"
  VehSpd/1 -> Scope/2, In-house CAVE/2(In2), PIF/2(In2), Predictive/2(In2)

== system CAVE_MachE_dSPACE_250912/Vehicle Under Test3/Vehicle/Front Wheel Drive/Ideal Diff/Power Bus ==
  DriveshftTrq : Inport
  Speed : Inport  Port=2
  Bus Creator : BusCreator  Inputs=1
  Bus Creator5 : BusCreator  Inputs=2
  Bus Creator6 : BusCreator  Inputs=3
  Bus Creator7 : BusCreator  Inputs=1
  Constant : Constant  Value=0
  Constant1 : Constant  Value=0
  Constant2 : Constant  Value=0
  Demux : Demux  Outputs=3
  Power Accounting Bus Creator : autolibpowerinfoutils/Power Accounting Bus Creator  AssctBlkSelPopup=Parent reference block  RefBlkName='autolibshareddiff/Open Differential'  PwrTrnsfrdCheckBox=on  PwrNotTrnsfrdCheckBox=on  PwrStoredCheckBox=on  aMode=aMode
  Signal Specification5 : SignalSpecification  Unit=W
  Transferred Power : Product
  Vector Concatenate : Concatenate  NumInputs=3
  PwrInfo : Outport
  wires:
  Bus Creator/1 -> Power Accounting Bus Creator/1
  Power Accounting Bus Creator/1 -> PwrInfo/1  "PwrInfo"
  Bus Creator5/1 -> Power Accounting Bus Creator/2
  Bus Creator6/1 -> Bus Creator/1  "PwrTrnsfrd"
  Transferred Power/1 -> Signal Specification5/1
  Signal Specification5/1 -> Vector Concatenate/3, Vector Concatenate/2, Vector Concatenate/1  "PwrDriveshft"
  Constant/1 -> Bus Creator5/1  "PwrMechLoss"
  Demux/3 -> Bus Creator6/3  "PwrAxl2"
  DriveshftTrq/1 -> Transferred Power/1
  Bus Creator7/1 -> Power Accounting Bus Creator/3
  Demux/2 -> Bus Creator6/2  "PwrAxl1"
  Demux/1 -> Bus Creator6/1  "PwrDriveshft"
  Speed/1 -> Transferred Power/2
  Vector Concatenate/1 -> Demux/1
  Constant1/1 -> Bus Creator5/2  "PwrDampLoss"
  Constant2/1 -> Bus Creator7/1  "PwrStoredShft"

== system CAVE_MachE_dSPACE_250912/Vehicle Under Test3/Vehicle/Front Wheel Drive/Ideal Diff AWD/Power Bus ==
  DriveshftTrq : Inport
  Speed : Inport  Port=2
  Bus Creator : BusCreator  Inputs=1
  Bus Creator5 : BusCreator  Inputs=2
  Bus Creator6 : BusCreator  Inputs=3
  Bus Creator7 : BusCreator  Inputs=1
  Constant : Constant  Value=0
  Constant1 : Constant  Value=0
  Constant2 : Constant  Value=0
  Demux : Demux  Outputs=3
  Power Accounting Bus Creator : autolibpowerinfoutils/Power Accounting Bus Creator  AssctBlkSelPopup=Parent reference block  RefBlkName='autolibshareddiff/Open Differential'  PwrTrnsfrdCheckBox=on  PwrNotTrnsfrdCheckBox=on  PwrStoredCheckBox=on  aMode=aMode
  Signal Specification5 : SignalSpecification  Unit=W
  Transferred Power : Product
  Vector Concatenate : Concatenate  NumInputs=3
  PwrInfo : Outport
  wires:
  Bus Creator/1 -> Power Accounting Bus Creator/1
  Power Accounting Bus Creator/1 -> PwrInfo/1  "PwrInfo"
  Bus Creator5/1 -> Power Accounting Bus Creator/2
  Bus Creator6/1 -> Bus Creator/1  "PwrTrnsfrd"
  Transferred Power/1 -> Signal Specification5/1
  Signal Specification5/1 -> Vector Concatenate/3, Vector Concatenate/2, Vector Concatenate/1  "PwrDriveshft"
  Constant/1 -> Bus Creator5/1  "PwrMechLoss"
  Demux/3 -> Bus Creator6/3  "PwrAxl2"
  DriveshftTrq/1 -> Transferred Power/1
  Bus Creator7/1 -> Power Accounting Bus Creator/3
  Demux/2 -> Bus Creator6/2  "PwrAxl1"
  Demux/1 -> Bus Creator6/1  "PwrDriveshft"
  Speed/1 -> Transferred Power/2
  Vector Concatenate/1 -> Demux/1
  Constant1/1 -> Bus Creator5/2  "PwrDampLoss"
  Constant2/1 -> Bus Creator7/1  "PwrStoredShft"

== system CAVE_MachE_dSPACE_250912/Vehicle Under Test3/Vehicle/Front Wheel Drive/Real Diff/Power Bus ==
  DriveshftTrq : Inport
  Speed : Inport  Port=2
  Bus Creator : BusCreator  Inputs=1
  Bus Creator5 : BusCreator  Inputs=2
  Bus Creator6 : BusCreator  Inputs=3
  Bus Creator7 : BusCreator  Inputs=1
  Constant : Constant  Value=0
  Constant1 : Constant  Value=0
  Constant2 : Constant  Value=0
  Demux : Demux  Outputs=3
  Power Accounting Bus Creator : autolibpowerinfoutils/Power Accounting Bus Creator  AssctBlkSelPopup=Parent reference block  RefBlkName='autolibshareddiff/Open Differential'  PwrTrnsfrdCheckBox=on  PwrNotTrnsfrdCheckBox=on  PwrStoredCheckBox=on  aMode=aMode
  Signal Specification5 : SignalSpecification  Unit=W
  Transferred Power : Product
  Vector Concatenate : Concatenate  NumInputs=3
  PwrInfo : Outport
  wires:
  Bus Creator/1 -> Power Accounting Bus Creator/1
  Power Accounting Bus Creator/1 -> PwrInfo/1  "PwrInfo"
  Bus Creator5/1 -> Power Accounting Bus Creator/2
  Bus Creator6/1 -> Bus Creator/1  "PwrTrnsfrd"
  Transferred Power/1 -> Signal Specification5/1
  Signal Specification5/1 -> Vector Concatenate/3, Vector Concatenate/2, Vector Concatenate/1  "PwrDriveshft"
  Constant/1 -> Bus Creator5/1  "PwrMechLoss"
  Demux/3 -> Bus Creator6/3  "PwrAxl2"
  DriveshftTrq/1 -> Transferred Power/1
  Bus Creator7/1 -> Power Accounting Bus Creator/3
  Demux/2 -> Bus Creator6/2  "PwrAxl1"
  Demux/1 -> Bus Creator6/1  "PwrDriveshft"
  Speed/1 -> Transferred Power/2
  Vector Concatenate/1 -> Demux/1
  Constant1/1 -> Bus Creator5/2  "PwrDampLoss"
  Constant2/1 -> Bus Creator7/1  "PwrStoredShft"

== system CAVE_MachE_dSPACE_250912/Vehicle Under Test3/Vehicle/Powertrain Supervisory Controller /Engine Torque Command/Accel Pedal to Traction Wheel Torque Request1 ==
  note: Convert Accelerator Pedal Position to Torque Command
      | using Motor Torque Speed Curve
  AccelPdl : Inport
  MotSpd : Inport  Port=2
  Max Motor Torque : Subsystem
  Product1 : Product
  TrqCmd : Outport  VectorParamsAs1DForOutWhenUnconnected=off
  wires:
  Max Motor Torque/1(MtrTrqMax) -> Product1/2
  MotSpd/1 -> Max Motor Torque/1(MtrSpd)
  AccelPdl/1 -> Product1/1
  Product1/1 -> TrqCmd/1

== system CAVE_MachE_dSPACE_250912/Vehicle Under Test3/Vehicle/Powertrain Supervisory Controller /Engine Torque Command/Battery Management System ==
  note: Behaviorial BMS System. Limits battery charge / discharge power based on SOC.
      |
      | Charge/Discharge Limits and curves can be adjusted if using a larger battery pack
      | or motor power is changed.
  SOC : Inport
  ChrgLmt : Lookup_n-D  NumberOfTableDimensions=1  BreakpointsForDimension1=BattChargeLimitSocBpts  Table=BattChargeLimitTbl  ExtrapMethod=Clip  UseLastTableValue=on  InternalRulePriority=Speed  RndMeth=Simplest
  DischrgLmt : Lookup_n-D  NumberOfTableDimensions=1  BreakpointsForDimension1=BattDischargeLimitSocBpts  Table=BattDischargeLimitTbl  ExtrapMethod=Clip  UseLastTableValue=on  InternalRulePriority=Speed  RndMeth=Simplest
  MaxChrg : Constant  Value=BattChargeLimitMaxPwr
  MaxDischrg : Constant  Value=BattDischargeMaxPwr
  Product : Product
  Product1 : Product
  BattPwrDischrgLmt : Outport  VectorParamsAs1DForOutWhenUnconnected=off
  BattPwrChrgLmt : Outport  Port=2  VectorParamsAs1DForOutWhenUnconnected=off
  wires:
  DischrgLmt/1 -> Product/1
  ChrgLmt/1 -> Product1/1
  Product1/1 -> BattPwrChrgLmt/1
  Product/1 -> BattPwrDischrgLmt/1
  MaxDischrg/1 -> Product/2
  MaxChrg/1 -> Product1/2
  SOC/1 -> ChrgLmt/1, DischrgLmt/1

== system CAVE_MachE_dSPACE_250912/Vehicle Under Test3/Vehicle/Powertrain Supervisory Controller /Engine Torque Command/Motor Torque Arbitration and Power Management ==
  MotTrqCmdTrac : Inport
  AccelPdl : Inport  Port=2
  BattPwrDisChrgLmt : Inport  Port=3
  "BattPwrChrgLmt " : Inport  Port=4
  MotSpd : Inport  Port=5
  MotTrqCmdRegen : Inport  Port=6
  Accel Decel Switch : Switch  Criteria=u2 > Threshold  SaturateOnIntegerOverflow=off  InputSameDT=off
  Compare To Constant : simulink/Logic and Bit Operations/Compare To Constant  relop=>  const=0  OutDataTypeStr=boolean
  Power Management : Subsystem
  MotTrqCmdFinal : Outport  VectorParamsAs1DForOutWhenUnconnected=off
  wires:
  Compare To Constant/1 -> Accel Decel Switch/2
  MotSpd/1 -> Power Management/3(MotSpd)
  "BattPwrChrgLmt "/1 -> Power Management/2(BattPwrChrgLmt)
  BattPwrDisChrgLmt/1 -> Power Management/1(BattPwrDischrgLmt)
  Accel Decel Switch/1 -> Power Management/4(MotTrqCmd)
  Power Management/1(MotTrqCmdFinal) -> MotTrqCmdFinal/1
  MotTrqCmdTrac/1 -> Accel Decel Switch/1
  MotTrqCmdRegen/1 -> Accel Decel Switch/3
  AccelPdl/1 -> Compare To Constant/1

== system CAVE_MachE_dSPACE_250912/Vehicle Under Test3/Vehicle/Powertrain Supervisory Controller /Engine Torque Command/Series Regen Braking ==
  note: These are all torque on wheels, which is DiffRatio*torque on motor
  note: - Total brake torque request based on brake pressure and parameters of disc brakes
      | - Use as much regenerative motor braking as possible
      | - Any braking torque request that cannot be provided by the motor, will be provided by the friction brakes
  BattSoc : Inport
  VehSpd : Inport  Port=2
  MotSpd : Inport  Port=3
  "DecelCmd " : Inport  Port=4
  ChrgLmt : Lookup_n-D  NumberOfTableDimensions=1  BreakpointsForDimension1=BattChargeLimitSocBpts  Table=BattChargeLimitTbl  ExtrapMethod=Clip  UseLastTableValue=on  InternalRulePriority=Speed  RndMeth=Simplest
  Gain : Gain  Gain=-1
  Gain1 : Gain  Gain=BrakeMaxTrq
  Gain2 : Gain  Gain=1/BrakeMaxTrq
  Max Motor Torque : LibPtSupervisoryCtrl/Powertrain Supervisory Controller /Engine Torque Command/Accel Pedal to Traction Wheel Torque Request/Max Motor Torque  SystemSampleTime=-1  VariantActivationTime=update diagram  AllowFlexibleInterface=on  Latency=0  AutoFrameSizeCalculation=off
  MinMax : MinMax  Inputs=2
  MotTrqReflectedToWheels : Gain  Gain=DiffRatio
  Product1 : Product
  Product3 : Product
  RegenBrakingCutoff : Lookup_n-D  NumberOfTableDimensions=1  BreakpointsForDimension1=SupvsryCtrlRegenSpdBpts  Table=SupvsryCtrlRegenBrkCutOffTbl  ExtrapMethod=Clip  UseLastTableValue=on  InternalRulePriority=Speed  RndMeth=Simplest
  Saturation : Saturate  UpperLimit=1  LowerLimit=0
  Saturation1 : Saturate  UpperLimit=1  LowerLimit=0
  Subtract : Sum  Inputs=+-
  WhlTrqReflectedToMot : Gain  Gain=1/DiffRatio
  " MotTrqCmdRegen" : Outport  VectorParamsAs1DForOutWhenUnconnected=off
  " BrkCmd" : Outport  Port=2  VectorParamsAs1DForOutWhenUnconnected=off
  wires:
  Gain2/1 -> Saturation1/1  "BrkTrqReqTotal"
  Subtract/1 -> Gain2/1
  Saturation/1 -> Gain1/1
  "DecelCmd "/1 -> Saturation/1  "BrkPrsReq"
  Gain/1 -> " MotTrqCmdRegen"/1  "MotTrqCmdRegen"
  WhlTrqReflectedToMot/1 -> Gain/1
  MotTrqReflectedToWheels/1 -> MinMax/2  "MotTrqMaxWhls"
  MotSpd/1 -> Max Motor Torque/1
  BattSoc/1 -> ChrgLmt/1
  Product1/1 -> Product3/2  "RegenFactor"
  RegenBrakingCutoff/1 -> Product1/1
  VehSpd/1 -> RegenBrakingCutoff/1
  ChrgLmt/1 -> Product1/2
  MinMax/1 -> Product3/1  "min"
  Max Motor Torque/1 -> MotTrqReflectedToWheels/1  "MotTrqMax"
  Saturation1/1 -> " BrkCmd"/1
  Product3/1 -> Subtract/2, WhlTrqReflectedToMot/1  "MotTrqRegenWhl"
  Gain1/1 -> MinMax/1, Subtract/1  "BrkTrqReqTotal"
